simulink library "INT_StSys_StrtBas"  (R2016b)
settings: Solver=VariableStepAuto  StartTime=0.0  StopTime=10.0  RelTol=1e-3
settings Model: Creator=Administrator  LastModifiedBy=Administrator

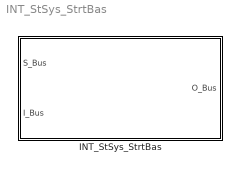
== system INT_StSys_StrtBas ==
  INT_StSys_StrtBas : Subsystem

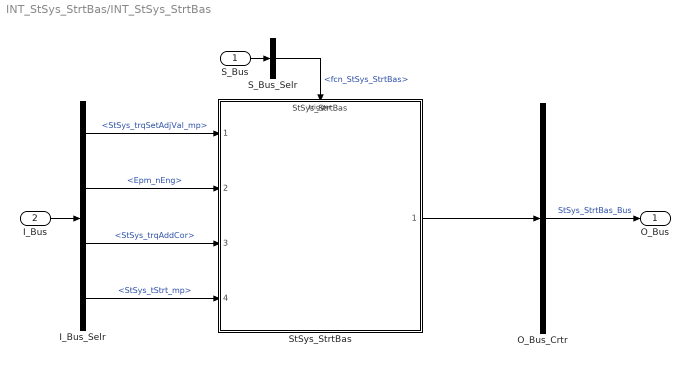
== system INT_StSys_StrtBas/INT_StSys_StrtBas ==
  S_Bus : Inport
  I_Bus : Inport  Port=2
  I_Bus_Selr : BusSelector  OutputSignals=StSys_trqSetAdjVal_mp,Epm_nEng,StSys_trqAddCor,StSys_tStrt_mp
  O_Bus_Crtr : BusCreator  Inputs=1
  S_Bus_Selr : BusSelector  OutputSignals=fcn_StSys_StrtBas
  StSys_StrtBas : ModelReference  ModelNameDialog=StSys_StrtBas  SimulationMode=Normal  ModelReferenceVersion=1.18  TriggerPortName=function  TriggerPortTriggerType=function-call  TriggerPortStatesWhenEnabling=held
  O_Bus : Outport
  wires:
  S_Bus_Selr/1 -> StSys_StrtBas/Trigger  "<fcn_StSys_StrtBas>"
  S_Bus/1 -> S_Bus_Selr/1
  I_Bus/1 -> I_Bus_Selr/1
  I_Bus_Selr/1 -> StSys_StrtBas/1  "<StSys_trqSetAdjVal_mp>"
  I_Bus_Selr/2 -> StSys_StrtBas/2  "<Epm_nEng>"
  I_Bus_Selr/3 -> StSys_StrtBas/3  "<StSys_trqAddCor>"
  I_Bus_Selr/4 -> StSys_StrtBas/4  "<StSys_tStrt_mp>"
  O_Bus_Crtr/1 -> O_Bus/1  "StSys_StrtBas_Bus"
  StSys_StrtBas/1 -> O_Bus_Crtr/1
